simulink library "Library_SII"  (R2018b)
settings: Solver=ode45  StartTime=0.0  StopTime=10.0  RelTol=1e-3  EnableMultiTasking=on
undefined symbols (not defined in the file or in its folder): coder, gcbh, r, simscape
libraries: fl_lib x156, nesl_utility x80, $bdroot x46, simulink x17, powerlib x12, mblibv1 x11, Simscape_SII_lib x11, elec_lib x10, Pneumatic_lib x4, peRmsMeasurement x1, powerlib_extras x1
(part 1 of 6)
settings Model: Creator=Cedrick  LastModifiedBy=Cedrick
settings DataIOCC: LimitDataPoints=on  SaveFormat=Array  SignalLoggingSaveFormat=ModelDataLogs
settings OptimizationCC: ExpressionDepthLimit=2147483647  LifeSpan=inf
settings DebuggingCC: UnderspecifiedInitializationDetection=Classic  MergeDetectMultiDrivingBlocksExec=none  SolverPrmCheckMsg=warning  FcnCallInpInsideContextMsg=warning  StateNameClashWarn=warning  SFUnexpectedBacktrackingDiag=warning  SFNoUnconditionalDefaultTransitionDiag=warning  SFExecutionAtInitializationDiag=none
settings HardwareCC: ProdBitPerPointer=32  ProdBitPerSizeT=32  ProdBitPerPtrDiffT=32  ProdLargestAtomicFloat=None  ProdIntDivRoundTo=Undefined  ProdEndianess=Unspecified  ProdWordSize=32  ProdHWDeviceType=32-bit Generic
settings ModelReferenceCC: PropagateSignalLabelsOutOfModel=off
settings SFSimCC: SimUseLocalCustomCode=off
settings RTWCC: RTWUseLocalCustomCode=off
settings CodeAppCC: StateflowObjectComments=on
settings GRTTargetCC: TargetLangStandard=C89/C90 (ANSI)  GeneratePreprocessorConditionals=Disable all  CombineOutputUpdateFcns=off  GRTInterface=on
settings ConfigComp: CovMetricSettings=dw  CovHtmlReporting=on  CovSaveCumulativeToWorkspaceVar=on  CovSaveSingleToWorkspaceVar=on  CovExternalEMLEnable=off  CovSFcnEnable=off

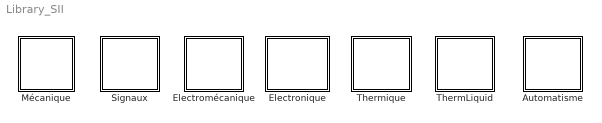
== system Library_SII ==
  Automatisme : Subsystem  AncestorBlock=Library_SII/ThermLiquid
      mask Display: image('Automatisme.bmp');
  Electromécanique : Subsystem
      mask Display: image(imread('Electromecanique.bmp'))
  Electronique : Subsystem
      mask Display: image(imread('Electronique.bmp'))
  Mécanique : Subsystem  mask(Mecanique){}
      mask Display: image('Mecanique.bmp');
  Signaux : Subsystem
      mask Display: image(imread('Signaux.bmp'))
  ThermLiquid : Subsystem
      mask Display: image('ThermLiquid.bmp')
  Thermique : Subsystem
      mask Display: image(imread('Thermique.bmp'))

== system Library_SII/Automatisme ==
  Vérin : Subsystem  mask(Vérin){T=3, N=10}
      mask prompts: T "Durée du mouvement"; N "Nombre de positions"
      mask help:
      | Permet de simuler le comportement simple d'un vérin pneumatique ou hydraulique, du point de vue partie commande.
      | Entrée : 0 = ordre de sortir ; 1 = ordre de rentrer
      | Sorties :
      |  - r = vérin rentré
      |  - s = vérin sorti
      |  - x = position du vérin (0 = rentré)
      |
      | Paramètres :
      |  - Durée du mouvement (s)
      |  - Nombre de positions
      mask Display:
      | plot([0 0.6 0.6 0 0],[0.4 0.4 0.6 0.6 0.4])
      | plot([0.6 0.7 0.7 0.6 0.6],[0.05 0.05 0.95 0.95 0.05])
      | color('blue')
      | plot([0.45 0.45 1 1 0.45 0.45],[0.35 0 0 1 1 0.65])
      | plot([0.35 0.55],[0.35 0.35])
      | plot([0.35 0.55],[0.65 0.65])

== system Library_SII/Electromécanique ==
  Commande moteur Position : Subsystem  AncestorBlock=|  mask(Commande de position moteur){Umax=5, e=1, P=100, I=1, D=0}
      | Library_SII/Electromécanique/Commande moteur
      | Position
      | (pour codeur incrémental)
      mask prompts: Umax "Tension maximum [V]"; e "Erreur tolérée [°]"
      mask help:
      | Asservissement en position d'un moteur à courant continu
      | piloté en tension.
      | En entrée :
      |  * cons pos : consigne de position angulaire (en °)
      |  * pos codeur : position mesurée (par un codeur)
      |
      | +mot et GND sont des ports physiques électriques pour alimenter le moteur.
      mask DialogControl Container4 Prompt: PID
  Décodeur pour codeur incrémental : Subsystem  mask(Commande de position moteur){r=1, inv=on}
      mask prompts: r "Résolution du codeur [°]"; inv "Inverser le sens"
      mask help:
      | Asservissement en position d'un moteur à courant continu
      | piloté en tension.
      | En entrée :
      |  * A et B : signaux issus d'un codeur incrémental
      |  * pos : consigne de position angulaire (en °)
      |
      | En sortie :
      |  * pos codeur : position calculée à partir des données du codeur
      |
      | +mot et GND sont des ports physiques électrique pour alimenter le moteur.
  Moteur CC (SPS-SM) : Subsystem  Tag=Moteur  Description=Moteur CC  mask(Moteur CC){axe=[1 0 0], R=0.989, L=0.0000718, K=1.39e-3, J=1.06e-6, kv=0.0002953, kc=0}
      mask prompts: axe "Vecteur directeur [x y z]"; R "Resistance (ohm)"; L "Inductance (H)"; K "Constante de vitesse (V/rpm)"; J "Inertie de l'arbre (kg.m^2)"; kv "Coefficient de frottement visqueux (N.m.s)"; kc "Coefficient de frottement sec"
      mask help:
      | Moteur à courant continu à aimants permanents.
      | L'axe du moteur est défini par le "Vecteur directeur"
      | et par la position du CS relié au stator.
      | Les autres paramètres sont fournis par les constructeurs de moteur.
      |
      | Les ports A+ et A- sont des ports physiques SimPowerSystems.
      | Les ports Stator et Rotor sont des ports mécaniques SimMechanics.
      mask Display:
      | image(imread('Motor.png'))
      | port_label('lconn', 1, 'Stator')
      | port_label('rconn', 1, 'Rotor')
      | port_label('lconn', 2, 'A+')
      | port_label('rconn', 2, 'A-')
  Moteur CC (SPS-SS) : Subsystem  Tag=Moteur  Description=Moteur CC  mask(Moteur CC){R=0.989, L=0.0000718, K=1.39e-3, J=1.06e-6, kv=0.0002953, kc=0}
      mask prompts: R "Resistance (ohm)"; L "Inductance (H)"; K "Constante de vitesse (V/rpm)"; J "Inertie de l'arbre (kg.m^2)"; kv "Coefficient de frottement visqueux (N.m.s)"; kc "Coefficient de frottement sec"
      mask help:
      | Moteur à courant continu à aimants permanents.
      | Les paramètres sont fournis par les constructeurs de moteur.
      |
      | Les ports A+ et A- sont des ports physiques SimPowerSystems.
      | Les ports Stator et Rotor sont des ports mécaniques SimScape.
      mask Display:
      | image(imread('Motor.png'))
      | port_label('lconn', 1, 'Stator')
      | port_label('rconn', 1, 'Rotor')
      | port_label('lconn', 2, 'A+')
      | port_label('rconn', 2, 'A-')
  Moteur PaP (SPS-SS) : Subsystem  Tag=Moteur  Description=Moteur PaP  mask(Moteur CC){R=0.989, L=0.0000718, K=1.39e-3, J=1.06e-6, kv=0.0002953, kc=0}
      mask prompts: R "Resistance (ohm)"; L "Inductance (H)"; K "Constante de vitesse (V/rpm)"; J "Inertie de l'arbre (kg.m^2)"; kv "Coefficient de frottement visqueux (N.m.s)"; kc "Coefficient de frottement sec"
      mask help:
      | Moteur à courant continu à aimants permanents.
      | Les paramètres sont fournis par les constructeurs de moteur.
      |
      | Les ports A+ et A- sont des ports physiques SimPowerSystems.
      | Les ports Stator et Rotor sont des ports mécaniques SimScape.
      mask Display:
      | image(imread('moteur_pap.jpg'))
      | port_label('lconn', 1, 'Stator')
      | port_label('rconn', 1, 'Rotor')
      | port_label('lconn', 2, 'A+')
      | port_label('rconn', 2, 'A-')
      | port_label('lconn', 3, 'B+')
      | port_label('rconn', 3, 'B-')
  Pont en H : Subsystem  mask(Pont en H){}
      mask help:
      | Mode de fonctionnement
      |  +1 : avant
      |  -1 : arrière
      |   0 : libre
      |   2 : freinage
  Servomoteur : Subsystem  mask(Servomoteur RC){U1=4.8, C1=0.33, d1=0.21, I1=0.15, I01=0.008, U2=6, C2=0.41, d2=0.16, I2=0.18, I02=0.0088, L=1e-5, P=30, I=2, D=0, res=1}
      mask prompts: U1 "Tension [V]"; C1 "Couple de calage [Nm]"; d1 "Vitesse à vide [s/60°]"; I1 "Courant à vide [A]"; I01 "Courant à l'arrêt [A]"; U2 "Tension [V]"; C2 "Couple de calage [Nm]"; d2 "Vitesse à vide [s/60°]"; I2 "Courant à vide [A]"; I02 "Courant à l'arrêt [A]"; L "Inductance moteur [H]"; res "Résolution capteur [°]"
      mask help:
      | Servomoteur de type modélisme.
      |
      | Deux ports physiques pour l'alimentation électrique.
      | (permet de mesurer des courants)
      | Un port Simulink pour la consigne angulaire (en degrés).
      |
      |
      | Caractéristiques par défaut : HITEC HS-422
      mask init:
      | w1 = pi/(3*d1); %rad/s
      | w2 = pi/(3*d2);
      | 
      | R01 = U1/I01;   % Ohm
      | R02 = U2/I02;
      | R0 = (R01+R02)/2;
      | 
      | I1 = I1-U1/R01;
      | I2 = I2-U2/R02;
      | 
      | delta = C1^2*w1^2+4*w1*I1*U1*C1;
      | K = (-C1*w1+sqrt(delta))/(2*w1*I1);
      | 
      | delta = C2^2*w2^2+4*w2*I2*U2*C2;
      | K = 0.5*(K + (-C2*w2+sqrt(delta))/(2*w2*I2));
      | 
      | R = (U1-K*w1)/I1;
      | R = 0.5*(R+(U2-K*w2)/I2);
      | 
      | kv = K*(I1-I2)/(w1-w2);
      | 
      | Cf = K*I1-kv*w1;
      | 
      | Cfc = K/R*U1 - C1;
      | Cfc = K/R*U2 - C2;
      mask DialogControl Container8 Prompt: Caractéristiques nominales
      mask DialogControl Container3 Prompt: Tension nominale 1
      mask DialogControl Container3_copy Prompt: Tension nominale 2
      mask DialogControl Container9 Prompt: PID
      mask DialogControl Container12 Prompt: Résolution
      mask Display:
      | image('servo.png')
      | port_label('input', 1, 'a [°]')
      | port_label('output', 1, 'w [°/s]')
      | port_label('output', 2, 'a [°]')
      | port_label('output', 3, 'Cm [Nm]')
  Servomoteur modèle de connaissance : Subsystem  mask(Servomoteur RC){L=1e-5, P=30, I=2, D=0, res=1}
      mask prompts: L "Inductance moteur [H]"; res "Résolution capteur [°]"
      mask help:
      | Servomoteur de type modélisme.
      |
      | Deux ports physiques pour l'alimentation électrique.
      | (permet de mesurer des courants)
      | Un port Simulink pour la consigne angulaire (en degrés).
      mask DialogControl Container8 Prompt: Caractéristiques nominales
      mask DialogControl Control2 Prompt: Modifier les paramètres à l'intérieur du bloc
      mask DialogControl Container9 Prompt: PID
      mask DialogControl Container12 Prompt: Résolution
      mask DialogControl Container11 Prompt: Tab
      mask Display:
      | image('servo.png')
      | port_label('input', 1, 'a [°]')
      | port_label('output', 1, 'w [°/s]')
      | port_label('output', 2, 'a [°]')
      | port_label('output', 3, 'C [Nm]')
  Servomoteur simple : Subsystem  AncestorBlock=Library_SII/Electromécanique/Servomoteur  mask(Servomoteur RC){U1=4.8, C1=0.33, d1=0.21, I1=0.15, I01=0.008, U2=6, C2=0.41, d2=0.16, I2=0.18, I02=0.0088, L=1e-5, P=30, I=2, D=0, res=1}
      mask prompts: U1 "Tension [V]"; C1 "Couple de calage [Nm]"; d1 "Vitesse à vide [s/60°]"; I1 "Courant à vide [A]"; I01 "Courant à l'arrêt [A]"; U2 "Tension [V]"; C2 "Couple de calage [Nm]"; d2 "Vitesse à vide [s/60°]"; I2 "Courant à vide [A]"; I02 "Courant à l'arrêt [A]"; L "Inductance moteur [H]"; res "Résolution capteur [°]"
      mask help:
      | Servomoteur de type modélisme.
      |
      | Deux ports physiques pour l'alimentation électrique.
      | (permet de mesurer des courants)
      | Un port Simulink pour la consigne angulaire (en degrés).
      |
      |
      | Caractéristiques par défaut : HITEC HS-422
      mask init: same as Library_SII/Electromécanique/Servomoteur
      mask DialogControl Container8 Prompt: Caractéristiques nominales
      mask DialogControl Container3 Prompt: Tension nominale 1
      mask DialogControl Container3_copy Prompt: Tension nominale 2
      mask DialogControl Container9 Prompt: PID
      mask DialogControl Container12 Prompt: Résolution
      mask Display:
      | image('servo.png')
      | port_label('input', 1, 'a [°]')
      | port_label('output', 1, 'w [°/s]')
      | port_label('output', 2, 'a [°]')
      | port_label('output', 3, 'Cm [Nm]')
  Servomoteur simple V1 : Subsystem  mask(Servomoteur RC){U1=4.8, C1=0.33, d1=0.21, I1=0.15, I01=0.008, U2=6, C2=0.41, d2=0.16, I2=0.18, I02=0.0088, L=1e-5, P=30, I=2, D=0}
      mask prompts: U1 "Tension [V]"; C1 "Couple de calage [Nm]"; d1 "Vitesse à vide [s/60°]"; I1 "Courant à vide [A]"; I01 "Courant à l'arrêt [A]"; U2 "Tension [V]"; C2 "Couple de calage [Nm]"; d2 "Vitesse à vide [s/60°]"; I2 "Courant à vide [A]"; I02 "Courant à l'arrêt [A]"; L "Inductance moteur [H]"
      mask help:
      | Servomoteur de type modélisme.
      |
      | Deux ports physiques pour l'alimentation électrique.
      | (permet de mesurer des courants)
      | Un port Simulink pour la consigne angulaire (en degrés).
      mask init:
      | w1 = pi/(3*d1); %rad/s
      | w2 = pi/(3*d2);
      | 
      | R01 = U1/I01;   % Ohm
      | R02 = U2/I02;
      | R0 = (R01+R02)/2;
      | 
      | I1 = I1-U1/R01;
      | I2 = I2-U2/R02;
      | 
      | %R = (U1*w2-U2*w1)/(I1*w2-I2*w1)
      | %R = (U1*C2-U2*C1)/(I1*C2-I2*C1)
      | %K = (U1-R*I1)/w1
      | %K = (C1/U1-C2/U2)/(I2/U2-I1/U1)
      | %K = (U1*I2-U2*I1)/(w1*I2-w2*I1)
      | %R = (U1-K*w1)/I1
      | %R = (U2-K*w2)/I2
      | 
      | 
      | delta = C1^2*w1^2+4*w1*I1*U1*C1;
      | K = (-C1*w1+sqrt(delta))/(2*w1*I1);
      | 
      | delta = C2^2*w2^2+4*w2*I2*U2*C2;
      | K = 0.5*(K + (-C2*w2+sqrt(delta))/(2*w2*I2));
      | 
      | R = (U1-K*w1)/I1;
      | R = 0.5*(R+(U2-K*w2)/I2);
      | 
      | kv = K*(I1-I2)/(w1-w2);
      | 
      | Cf = K*I1-kv*w1;
      | 
      | Cfc = K/R*U1 - C1;
      | Cfc = K/R*U2 - C2;
      mask DialogControl Container8 Prompt: Caractéristiques nominales
      mask DialogControl Container3 Prompt: Tension nominale 1
      mask DialogControl Container3_copy Prompt: Tension nominale 2
      mask DialogControl Container9 Prompt: PID
      mask Display:
      | image('servo.png')
      | port_label('input', 1, 'a [°]')
      | port_label('output', 1, 'w [°/s]')
      | port_label('output', 2, 'a [°]')
      | port_label('output', 3, 'C [Nm]')

== system Library_SII/Electronique ==
  Ampèremètre : Subsystem  mask(Ampèremètre){}
      mask help: Ampèremètre avec un signal de sortie au format Simulink
      mask Display:
      | plot([184.371736831963;184.043550999396;183.062154110669;181.436997554304;179.183732476342;176.324059051243;172.885517497347;168.901222849516;164.409546043246;159.453744381582;154.081544943642;148.344684946756;142.298413488781;136.000959469086;129.512970812418;122.896930396238;116.216554306448;109.536178216657;102.920137800477;96.4321491438092;90.134695124114;84.0884236661391;78.3515636692533;72.979364231313;68.0235625696485;63.5318857633786;59.5475911155478;56.1090495616519;53.2493761365527;50.9961110585907;49.3709545022264;48.3895576134986;48.0613717809319;48.3895576134986;49.3709545022264;50.9961110585907;53.2493761365528;56.109049561652;59.547591115548;63.5318857633788;68.0235625696487;72.9793642313131;78.3515636692534;84.0884236661394;90.1346951241142;96.4321491438093;102.920137800477;109.536178216657;116.216554306448;122.896930396238;129.512970812418;136.000959469086;142.298413488781;148.344684946756;154.081544943642;159.453744381582;164.409546043246;168.901222849516;172.885517497347;176.324059051243;179.183732476342;181.436997554304;183.062154110669;184.043550999396;184.371736831963;184.371736831963], [130.389304831624;123.708928741834;117.092888325653;110.604899668986;104.307445649291;98.2611741913157;92.5243141944298;87.1521147564895;82.1963130948251;77.7046362885552;73.7203416407244;70.2818000868285;67.4221266617293;65.1688615837672;63.5437050274029;62.5623081386751;62.2341223061085;62.5623081386751;63.5437050274029;65.1688615837672;67.4221266617293;70.2818000868285;73.7203416407244;77.7046362885552;82.1963130948251;87.1521147564896;92.5243141944299;98.2611741913158;104.307445649291;110.604899668986;117.092888325653;123.708928741834;130.389304831624;137.069680921414;143.685721337595;150.173709994262;156.471164013958;162.517435471932;168.254295468818;173.626494906759;178.582296568423;183.073973374693;187.058268022524;190.49680957642;193.356483001519;195.609748079481;197.234904635845;198.216301524573;198.54448735714;198.216301524573;197.234904635845;195.609748079481;193.356483001519;190.49680957642;187.058268022524;183.073973374693;178.582296568423;173.626494906759;168.254295468818;162.517435471933;156.471164013958;150.173709994263;143.685721337595;137.069680921415;130.389304831624;130.389304831624])
      | plot([0;240.936758928001;240.936758928001;0;0], [255.109509453177;255.109509453177;0;0;255.109509453177])
      | plot([134.798604995012;113.382004201412], [102.043803781271;158.734805881977])
      | plot([113.696954213083;92.9102534428239], [158.419855870306;102.043803781271])
      | plot([143.617205321789;124.720204621553], [102.043803781271;102.043803781271])
      | plot([101.41390375793;84.406603127718], [102.043803781271;102.043803781271])
      | plot([99.2092536762357;127.554754726589], [119.051104411483;119.051104411483])
      | plot([48.1873517856002;0], [130.389304831624;130.389304831624])
      | plot([184.245756827295;212.591257877648;212.591257877648;240.936758928001], [130.389304831624;130.389304831624;65.194652415812;65.194652415812])
      | ;
      | color('red');
      | port_label('output', 1,'I')
      | port_label('LConn', 1,'+')
      | port_label('RConn', 1,'-')
  Bobine entrée : Subsystem  mask{N=30, s=1e-6, D=0.1, l=0.01}
      mask prompts: N "Nombre de tours"; s "Section du fil [m²]"; D "Diamètre de la bobine [m]"; l "Longueur de la bobine [m]"
      mask init:
      | % Perméabilité magnétique du vide
      | mu0 = pi*4e-7;
      | 
      | % Résistivité cuivre
      | rho = 1.7e-8; % Ohm.m
      mask DialogControl s Tooltip: Section du fil constituant la bobine
  Cellule Photovoltaique SPS : Subsystem  mask(Cellule Photovoltaique SPS){Voc=0.6, Isc=5, Tjref=25, alpha=3.4e-4, TXI=3, EG=1.11, Rs=0.01, Rsh=50, Eref=1000, N=1.5}
      mask prompts: Voc "Tension à vide (V)"; Isc "Courant de court circuit (A)"; Tjref "Temperature de référence (°C)"; alpha "Coef de courant en température (°C^-1)"; TXI "Coef d'influence de la T°"; EG "Energie d'activation (eV)"; Rs "Résistance interne (Ohms)"; Rsh "Résistance de shunt (Ohm)"; Eref "Ensoleillement de référence (W/m²)"; N "Facteur de qualité"
      mask help:
      | Modèle d'une cellule photovoltaique.
      | En entrée :
      |   Ta : Température ambiante (°C)
      |   Ir : Irradiation (W/m²)
      |
      | En sortie :
      |   Ports physiques SimPowerSystems
      mask init:
      | % Charge de l'electron
      | q = 1.602e-19; % C
      | % Constante de Boltzmann
      | k = 1.38e-23;
      | % Degrés --> Kelvin
      | Kel = 273.15;
      | 
      | qkT = q/(k*(Tjref+Kel)); % 38.9358 à 25°C
      | 
      | % Courant de saturation de la diode (A)
      | % pour I = 0 (circuit ouvert)
      | I0d = ((Voc+Rs*Isc)/Rsh-Isc)/(exp(qkT*Rs*Isc/N)-exp(qkT*Voc/N));
      | 
      | % Courant de référence (A)
      | % pour U = 0 (court circuit)
      | I0 = Isc*(1+Rs/Rsh)+I0d*(exp(qkT*Rs*Isc/N)-1);
      | 
      | % Coef de tension en température (influe sur Iph)
      | beta = -2.17e-3; % mV/°C
      mask Display:
      | image(imread('cellulePV_poly.jpg'))
      | port_label('input', 1, 'Ta')
      | port_label('input', 2, 'Ir')
      | port_label('rconn', 1, '+')
      | port_label('rconn', 2, '-')
  Cellule Photovoltaique avec capteurs U et I SimElectronics : Subsystem  mask(Cellule Photovoltaique (SimElectronics)){typcell=polycristallin, Icc=4.5, Vco=0.601, Tcell=25, shunt=0, mesure=off, IRef=1000, TRef=25, Qf=1.4}
      mask prompts: typcell "Type"; Icc "Courant de court-circuit (A)"; Vco "Tension de circuit ouvert (V)"; Tcell "Température de cellule (°C)"; shunt "Shunter"; mesure "Mesurer le courant et la tension"; IRef "Irradiance de référence (W/m²)"; TRef "Température de référence (°C)"; Qf "Facteur de qualité"
      mask help:
      | Modèle d'une cellule photovoltaique.
      |  - mesure courant/tension
      |  - possibilité de shunter la cellule (par programmation)
      |
      | En entrée :
      |   Ir : Irradiation (W/m²)
      |
      | Connectique : ports physiques SimElectronics
      |
      | Caractéristiques :
      |     Courant de court-circuit (A)
      |     Tension de circuit ouvert (V)
      |     Température (°C) et irradiance (W/m²) de référence
      |
      | Température
      |     Température de cellule (°C)
      |
      | Il est possible de "tester" cette cellule grâce à l'interface graphique "CellulePV_IHM".
      |
      | Voir aussi la classe "pnl_etat_cellule.m" pour la programmation d'IHM.
      mask TypeOptions typcell: monocristallin | polycristallin | amorphe
      mask Callback typcell:
      | t = get_param(gcb, 'typcell');
      | switch t
      |     case 'monocristallin'
      |         n = '1.4';
      |     case 'polycristallin'
      |         n = '2';
      |     case 'amorphe'
      |         n = '10';
      | end
      | set_param(gcb, 'Qf', n)
      mask Display:
      | t = get_param(gcb, 'typcell');
      | switch t
      |     case 'monocristallin'
      |         image(imread('cellulePV_mono.jpg'))
      |     case 'polycristallin'
      |         image(imread('cellulePV_poly.jpg'))
      |     case 'amorphe'
      |         image(imread('cellulePV_amorphe.jpg'))
      | end
      | 
      | port_label('input', 1, 'Ir')
      | port_label('rconn', 1, '+')
      | port_label('rconn', 2, '-')
      | port_label('output', 1, 'I')
      | port_label('output', 2, 'U')
  Diode : Subsystem  mask(Diode){I0d=1e-6, N=1.5}
      mask prompts: I0d "Courant de saturation (A)"; N "Facteur de qualité"
      mask help:
      | Diode selon le modèle de Shockley :
      | Id = Is*(exp(Vd/(N*Vt))-1)
      |     avec Vt = k*Tj/q
      |
      |     Id : courant traversant la diode
      |     Vd : tension aux bornes de la diode
      |
      |     k : constante de Boltzmann
      |     q : charge de l'electron
      |
      | La température de jonction Tj (K) est donnée par le port Simulink Tj.
      |
      | Les paramètres intrinsèques à la diode sont :
      |     N : facteur de qualité (entre 1 et 2 pour les diodes en silicium)
      |     Id : courant de saturation de la diode (A)
      |
      | Les bornes A et C correspondent à l'anode et à la cathode de la diode.
      mask init:
      | % Charge de l'electron
      | q = 1.602e-19; % C
      | % Constante de Boltzmann
      | k = 1.38e-23;
      | % Degrés --> Kelvin
      | Kel = 273.15;
      | 
      | Tj = 300;
      mask Display:
      | image(imread('Diode.png'))
      | port_label('lconn', 1, 'A')
      | port_label('rconn', 1, 'C')
      | port_label('input', 1, 'Tj')
  Hacheur (PWM) : Subsystem  mask{f=500, A=12}
      mask prompts: f "Fréquence (Hz)"; A "Amplitude (V)"
  Hacheur (PWM) Tension variable : Subsystem  mask{f=500, A=12}
      mask prompts: f "Fréquence (Hz)"; A "Amplitude (V)"
  Interrupteur : Subsystem  mask(Interrupteur){}
      mask help: Interrupteur avec signal de commutation au format Simulink
      mask Display:
      | patch([178.308949107304;178.270428219378;178.155236532808;177.964483406507;177.700005897356;177.364351068347;176.960751458971;176.493093954097;175.965882351142;175.384193986049;174.753630835755;174.080265568098;173.370583058705;172.631417938094;171.869888770445;171.093329497935;170.309218810871;169.525108123807;168.748548851298;167.987019683648;167.247854563037;166.538172053645;165.864806785988;165.234243635694;164.6525552706;164.125343667646;163.657686162771;163.254086553395;162.918431724386;162.653954215236;162.463201088934;162.348009402364;162.309488514438;162.348009402364;162.463201088934;162.653954215236;162.918431724386;163.254086553395;163.657686162771;164.125343667646;164.6525552706;165.234243635694;165.864806785988;166.538172053645;167.247854563037;167.987019683648;168.748548851298;169.525108123807;170.309218810871;171.093329497935;171.869888770445;172.631417938094;173.370583058705;174.080265568098;174.753630835754;175.384193986049;175.965882351142;176.493093954096;176.960751458971;177.364351068347;177.700005897356;177.964483406507;178.155236532808;178.270428219378;178.308949107304;178.308949107304], [113.618216710165;112.834106023101;112.057546750592;111.296017582942;110.556852462331;109.847169952939;109.173804685282;108.543241534988;107.961553169894;107.43434156694;106.966684062065;106.563084452689;106.22742962368;105.962952114529;105.772198988228;105.657007301658;105.618486413732;105.657007301658;105.772198988228;105.962952114529;106.22742962368;106.563084452689;106.966684062065;107.43434156694;107.961553169894;108.543241534988;109.173804685282;109.847169952939;110.556852462331;111.296017582942;112.057546750592;112.834106023101;113.618216710165;114.402327397229;115.178886669738;115.940415837388;116.679580957999;117.389263467392;118.062628735048;118.693191885343;119.274880250436;119.80209185339;120.269749358265;120.673348967641;121.00900379665;121.273481305801;121.464234432102;121.579426118672;121.617947006598;121.579426118672;121.464234432102;121.273481305801;121.00900379665;120.673348967641;120.269749358265;119.80209185339;119.274880250436;118.693191885343;118.062628735048;117.389263467392;116.679580957999;115.940415837388;115.178886669738;114.402327397229;113.618216710165;113.618216710165], [0;0;0])
      | plot([178.308949107304;178.270428219378;178.155236532808;177.964483406507;177.700005897356;177.364351068347;176.960751458971;176.493093954097;175.965882351142;175.384193986049;174.753630835755;174.080265568098;173.370583058705;172.631417938094;171.869888770445;171.093329497935;170.309218810871;169.525108123807;168.748548851298;167.987019683648;167.247854563037;166.538172053645;165.864806785988;165.234243635694;164.6525552706;164.125343667646;163.657686162771;163.254086553395;162.918431724386;162.653954215236;162.463201088934;162.348009402364;162.309488514438;162.348009402364;162.463201088934;162.653954215236;162.918431724386;163.254086553395;163.657686162771;164.125343667646;164.6525552706;165.234243635694;165.864806785988;166.538172053645;167.247854563037;167.987019683648;168.748548851298;169.525108123807;170.309218810871;171.093329497935;171.869888770445;172.631417938094;173.370583058705;174.080265568098;174.753630835754;175.384193986049;175.965882351142;176.493093954096;176.960751458971;177.364351068347;177.700005897356;177.964483406507;178.155236532808;178.270428219378;178.308949107304;178.308949107304], [113.618216710165;112.834106023101;112.057546750592;111.296017582942;110.556852462331;109.847169952939;109.173804685282;108.543241534988;107.961553169894;107.43434156694;106.966684062065;106.563084452689;106.22742962368;105.962952114529;105.772198988228;105.657007301658;105.618486413732;105.657007301658;105.772198988228;105.962952114529;106.22742962368;106.563084452689;106.966684062065;107.43434156694;107.961553169894;108.543241534988;109.173804685282;109.847169952939;110.556852462331;111.296017582942;112.057546750592;112.834106023101;113.618216710165;114.402327397229;115.178886669738;115.940415837388;116.679580957999;117.389263467392;118.062628735048;118.693191885343;119.274880250436;119.80209185339;120.269749358265;120.673348967641;121.00900379665;121.273481305801;121.464234432102;121.579426118672;121.617947006598;121.579426118672;121.464234432102;121.273481305801;121.00900379665;120.673348967641;120.269749358265;119.80209185339;119.274880250436;118.693191885343;118.062628735048;117.389263467392;116.679580957999;115.940415837388;115.178886669738;114.402327397229;113.618216710165;113.618216710165])
      | patch([64.926944905892;64.888424017966;64.7732323313963;64.5824792050947;64.3180016959439;63.9823468669351;63.5787472575591;63.1110897526843;62.5838781497303;62.0021897846366;61.3716266343423;60.6982613666856;59.988578857293;59.2494137366818;58.4878845690323;57.7113252965232;56.927214609459;56.1431039223949;55.3665446498857;54.6050154822362;53.8658503616251;53.1561678522324;52.4828025845758;51.8522394342815;51.2705510691878;50.7433394662337;50.275681961359;49.872082351983;49.5364275229742;49.2719500138234;49.0811968875218;48.9660052009521;48.9274843130261;48.9660052009521;49.0811968875218;49.2719500138234;49.5364275229742;49.8720823519831;50.275681961359;50.7433394662338;51.2705510691878;51.8522394342816;52.4828025845758;53.1561678522325;53.8658503616251;54.6050154822362;55.3665446498858;56.143103922395;56.927214609459;57.7113252965232;58.4878845690323;59.2494137366818;59.988578857293;60.6982613666856;61.3716266343422;62.0021897846366;62.5838781497303;63.1110897526843;63.5787472575591;63.982346866935;64.3180016959439;64.5824792050947;64.7732323313963;64.888424017966;64.926944905892;64.926944905892], [113.618216710165;112.834106023101;112.057546750592;111.296017582942;110.556852462331;109.847169952939;109.173804685282;108.543241534988;107.961553169894;107.43434156694;106.966684062065;106.563084452689;106.22742962368;105.962952114529;105.772198988228;105.657007301658;105.618486413732;105.657007301658;105.772198988228;105.962952114529;106.22742962368;106.563084452689;106.966684062065;107.43434156694;107.961553169894;108.543241534988;109.173804685282;109.847169952939;110.556852462331;111.296017582942;112.057546750592;112.834106023101;113.618216710165;114.402327397229;115.178886669738;115.940415837388;116.679580957999;117.389263467392;118.062628735048;118.693191885343;119.274880250436;119.80209185339;120.269749358265;120.673348967641;121.00900379665;121.273481305801;121.464234432102;121.579426118672;121.617947006598;121.579426118672;121.464234432102;121.273481305801;121.00900379665;120.673348967641;120.269749358265;119.80209185339;119.274880250436;118.693191885343;118.062628735048;117.389263467392;116.679580957999;115.940415837388;115.178886669738;114.402327397229;113.618216710165;113.618216710165], [0;0;0])
      | plot([64.926944905892;64.888424017966;64.7732323313963;64.5824792050947;64.3180016959439;63.9823468669351;63.5787472575591;63.1110897526843;62.5838781497303;62.0021897846366;61.3716266343423;60.6982613666856;59.988578857293;59.2494137366818;58.4878845690323;57.7113252965232;56.927214609459;56.1431039223949;55.3665446498857;54.6050154822362;53.8658503616251;53.1561678522324;52.4828025845758;51.8522394342815;51.2705510691878;50.7433394662337;50.275681961359;49.872082351983;49.5364275229742;49.2719500138234;49.0811968875218;48.9660052009521;48.9274843130261;48.9660052009521;49.0811968875218;49.2719500138234;49.5364275229742;49.8720823519831;50.275681961359;50.7433394662338;51.2705510691878;51.8522394342816;52.4828025845758;53.1561678522325;53.8658503616251;54.6050154822362;55.3665446498858;56.143103922395;56.927214609459;57.7113252965232;58.4878845690323;59.2494137366818;59.988578857293;60.6982613666856;61.3716266343422;62.0021897846366;62.5838781497303;63.1110897526843;63.5787472575591;63.982346866935;64.3180016959439;64.5824792050947;64.7732323313963;64.888424017966;64.926944905892;64.926944905892], [113.618216710165;112.834106023101;112.057546750592;111.296017582942;110.556852462331;109.847169952939;109.173804685282;108.543241534988;107.961553169894;107.43434156694;106.966684062065;106.563084452689;106.22742962368;105.962952114529;105.772198988228;105.657007301658;105.618486413732;105.657007301658;105.772198988228;105.962952114529;106.22742962368;106.563084452689;106.966684062065;107.43434156694;107.961553169894;108.543241534988;109.173804685282;109.847169952939;110.556852462331;111.296017582942;112.057546750592;112.834106023101;113.618216710165;114.402327397229;115.178886669738;115.940415837388;116.679580957999;117.389263467392;118.062628735048;118.693191885343;119.274880250436;119.80209185339;120.269749358265;120.673348967641;121.00900379665;121.273481305801;121.464234432102;121.579426118672;121.617947006598;121.579426118672;121.464234432102;121.273481305801;121.00900379665;120.673348967641;120.269749358265;119.80209185339;119.274880250436;118.693191885343;118.062628735048;117.389263467392;116.679580957999;115.940415837388;115.178886669738;114.402327397229;113.618216710165;113.618216710165])
      | plot([56.927214609459;161.805568495765], [113.618216710165;56.927214609459])
      | plot([227.000220911577;113.618216710165;113.618216710165], [170.309218810871;170.309218810871;82.4381655547768])
      | patch([0;227.23643342033;227.23643342033;0;0;0.472425017505884;0.472425017505884;226.764008402824;226.764008402824;0.472425017505884;0], [227.23643342033;227.23643342033;0;0;227.23643342033;226.764008402824;0.472425017505884;0.472425017505884;226.764008402824;226.764008402824;227.23643342033], [1;1;1])
      | plot([170.309218810871;198.654719861224;198.654719861224;227.000220911577], [113.618216710165;113.618216710165;56.927214609459;56.927214609459])
      | plot([56.927214609459;0.236212508752942], [113.618216710165;113.618216710165])
      | ;
      | color('red');
      | port_label('LConn', 1,'')
      | port_label('RConn', 1,'')
  Mesure Puissance RMS : Subsystem  mask(Mesure de puissance Electrique RMS){ff=50}
      mask prompts: ff "Fréquence fondamentale [Hz]"
      mask help:
      | Mesure le courant, la tension et la puissance RMS sur un circuit.
      | Retourne les valeurs sous forme d'un vecteur [I, U, P]
      mask init:
      | fs = get_param(bdroot, 'FixedStep');
      | 
      | % Longueur de la fenêtre de mesure RMS
      | lw = int32(ff*fs)
      mask Display: disp('RMS')
  Panneau photovoltaique SimElectronics : Subsystem  mask(Panneau Photovoltaïque (SimElectronics)){typcell=polycristallin, s=8, Icc=4.5, Vco=0.601, Tcell=30, C=[2.1         3.1         3.2], D=[0  50  50], shunt_diode=[1 1 1 1]}
      mask prompts: typcell "Type"; s "Nombre de cellules en série (x4)"; Icc "Courant de court-circuit (A)"; Vco "Tension de circuit ouvert (V)"; Tcell "Température de cellule (°C)"; C "Cellules occultées"; D "Degré d'occultation (%)"; shunt_diode "shunt diode"
      mask help:
      | Panneau Photovoltaïque 12V maxi
      |  - au maximum 4 rangées de 9 cellules occultables partiellement
      |  - possibilité de desactiver (shunter) les cellules par rangées de 4
      |  - possibilité d'utiliser ou non des diodes ByPass.
      |
      | Les caractéristiques Vco, et Icc des cellulles sont données pour les
      | valeurs de référence Tref = 25°C et Iref = 1000W/m².
      |
      | Entrées :
      |   Ir : Irradiance W/m²
      |
      | Sorties (3 vecteurs) :
      |   Ui : tensions aux bornes des cellules
      |   Ii : courants traversant les cellules
      |   Id : courants traversant les diodes de shunt
      |
      | Connectique : SimElectronics
      |
      | Pour gérer ce bloc, il est conseillé d'utiliser l'interface graphique "ModulePV_IHM.m".
      |
      | Voir aussi la classe "pnl_etat_module.m" pour la programmation d'IHM.
      mask init:
      | % Liste des valeurs degré d'occultation
      | % (1 pour toutes par défaut)
      | G = ones(4,9);
      | for l = 1:4
      |     for c = 1:9
      |         lc = l+c/10;
      |         G(l,c) = 1;
      |         for o = 1:length(C)
      |             if C(o) == lc
      |                 G(l,c) = D(o)/100;
      |             end
      |         end
      |     end
      | end
      | 
      | 
      | % Réalisation de la structure
      | for i = 1:9
      |     if i <= s
      |         v = '0';
      |     else
      |         v = '1';
      |     end
      |     for cell = 1:4
      |         ncell = [gcb, '/Cellule ', num2str(cell), '.', num2str(i)];
      |         set_param(ncell, 'shunt', v)
      |     end
      | end
      mask TypeOptions typcell: monocristallin | polycristallin | amorphe
      mask Callback typcell:
      | t = get_param(gcb, 'typcell');
      | c = find_system(gcb, 'Regexp', 'on', 'LookUnderMasks', 'all',...
      |     'FollowLinks', 'on', 'Name', 'Cellule+');
      | n = length(c);
      | for i = 1:n
      |     a = c{i,1};
      |     set_param(a, 'typcell', t )
      | end
      mask Callback D:
      | D = str2num(get_param(gcb, 'D'));
      | for d = 1:length(D)
      |     if D(d) > 100
      |         error('Le degré d''occultation doit être compris entre 0% et 100%')
      |     end
      | end
      mask Display:
      | image(imread('modulePV.png'))
      | port_label('input', 1, 'Ir')
      | port_label('rconn', 1, '+')
      | port_label('rconn', 2, '-')
      | port_label('output', 1, 'Ui')
      | port_label('output', 2, 'Ii')
      | port_label('output', 3, 'Id')
  Photorésistance : Subsystem  mask(Photorésistance){a=-4/5, b=-4/5+6}
      mask help:
      | Modèle :
      | log(R) = a log(E) + b
      | avec :
      |   - E : éclairement en lux
      |   - R : résistance en Ohm
      mask DialogControl ParameterGroupVar Prompt: Paramètres
      mask Display: image('images/photoresistance.png')
  Puissance-mètre : Subsystem
      mask Display:
      | x = [0.8, 0.796, 0.785, 0.767, 0.743, 0.712, 0.676, 0.636, 0.593, 0.547, 0.5, 0.453, 0.407, 0.364, 0.324, 0.288, 0.257, 0.233, 0.215, 0.204, 0.2, 0.204, 0.215, 0.233, 0.257, 0.288, 0.324, 0.364, 0.407, 0.453, 0.5, 0.547, 0.593, 0.636, 0.676, 0.712, 0.743, 0.767, 0.785, 0.796, 0.8];
      | y = [0.5, 0.563, 0.624, 0.682, 0.735, 0.783, 0.824, 0.856, 0.88, 0.895, 0.9, 0.895, 0.88, 0.856, 0.824, 0.783, 0.735, 0.682, 0.624, 0.563, 0.5, 0.437, 0.376, 0.318, 0.265, 0.217, 0.176, 0.144, 0.12, 0.105, 0.1, 0.105, 0.12, 0.144, 0.176, 0.217, 0.265, 0.318, 0.376, 0.437, 0.5];
      | plot(x, y);
      | color('red');
      | port_label('LConn', 1,'E+')
      | port_label('RConn', 1,'S+')
      | port_label('LConn', 2,'-')
  Simscape<->SPS : Subsystem  mask(Convertisseur Simscape SimPowerSystems){}
      mask help:
      | Convertisseur Simscape SimPowerSystems
      |
      | Attention : à utiliser avec prudence : créé des "algebraic loops"
      | web([docroot '/toolbox/simulink/ug/f7-8243.html#f7-19688'])
  Transformateur variable : Simscape_SII_lib/Ideal Transformer  i1_specify=off  i1_priority=High  i1=0 A  i1_nominal_specify=off  i1_nominal_unit=A  i1_nominal_value=1  v1_specify=off  v1_priority=High  v1=0 V  v1_nominal_specify=off  v1_nominal_unit=V  v1_nominal_value=1  i2_specify=off  i2_priority=High  i2=0 A  i2_nominal_specify=off  i2_nominal_unit=A  i2_nominal_value=1  v2_specify=off  v2_priority=High  v2=0 V  v2_nominal_specify=off  v2_nominal_unit=V  v2_nominal_value=1
  Voltmètre : Subsystem  mask(Voltmètre){}
      mask help: Voltmètre avec un signal de sortie au format Simulink
      mask Display:
      | plot([90.7056033611298;147.396605461836], [106.138153932989;127.554754726589])
      | plot([147.081655450165;90.7056033611298], [127.239804714918;148.026505485177])
      | plot([90.7056033611298;90.7056033611298], [97.3195536062121;116.216554306448])
      | plot([90.7056033611298;90.7056033611298], [139.522855170071;156.530155800283])
      | plot([184.371736831963;184.043550999396;183.062154110669;181.436997554304;179.183732476342;176.324059051243;172.885517497347;168.901222849516;164.409546043246;159.453744381582;154.081544943642;148.344684946756;142.298413488781;136.000959469086;129.512970812418;122.896930396238;116.216554306448;109.536178216657;102.920137800477;96.4321491438092;90.134695124114;84.0884236661391;78.3515636692533;72.979364231313;68.0235625696485;63.5318857633786;59.5475911155478;56.1090495616519;53.2493761365527;50.9961110585907;49.3709545022264;48.3895576134986;48.0613717809319;48.3895576134986;49.3709545022264;50.9961110585907;53.2493761365528;56.109049561652;59.547591115548;63.5318857633788;68.0235625696487;72.9793642313131;78.3515636692534;84.0884236661394;90.1346951241142;96.4321491438093;102.920137800477;109.536178216657;116.216554306448;122.896930396238;129.512970812418;136.000959469086;142.298413488781;148.344684946756;154.081544943642;159.453744381582;164.409546043246;168.901222849516;172.885517497347;176.324059051243;179.183732476342;181.436997554304;183.062154110669;184.043550999396;184.371736831963;184.371736831963], [130.389304831624;123.708928741834;117.092888325653;110.604899668986;104.307445649291;98.2611741913157;92.5243141944298;87.1521147564895;82.1963130948251;77.7046362885552;73.7203416407244;70.2818000868285;67.4221266617293;65.1688615837672;63.5437050274029;62.5623081386751;62.2341223061085;62.5623081386751;63.5437050274029;65.1688615837672;67.4221266617293;70.2818000868285;73.7203416407244;77.7046362885552;82.1963130948251;87.1521147564896;92.5243141944299;98.2611741913158;104.307445649291;110.604899668986;117.092888325653;123.708928741834;130.389304831624;137.069680921414;143.685721337595;150.173709994262;156.471164013958;162.517435471932;168.254295468818;173.626494906759;178.582296568423;183.073973374693;187.058268022524;190.49680957642;193.356483001519;195.609748079481;197.234904635845;198.216301524573;198.54448735714;198.216301524573;197.234904635845;195.609748079481;193.356483001519;190.49680957642;187.058268022524;183.073973374693;178.582296568423;173.626494906759;168.254295468818;162.517435471933;156.471164013958;150.173709994263;143.685721337595;137.069680921415;130.389304831624;130.389304831624])
      | plot([0;240.936758928001;240.936758928001;0;0], [255.109509453177;255.109509453177;0;0;255.109509453177])
      | plot([48.1873517856002;0], [130.389304831624;130.389304831624])
      | plot([184.245756827295;212.591257877648;212.591257877648;240.936758928001], [130.389304831624;130.389304831624;62.3601023107767;62.3601023107767])
      | ;
      | color('red');
      | port_label('output', 1,'V')
      | port_label('LConn', 1,'+')
      | port_label('RConn', 1,'-')
